simulink model "CustomTelemPX4"  (R2021a)
settings: Solver=FixedStepAuto  StartTime=0.0  StopTime=inf  RelTol=1e-3  EnableMultiTasking=on
InitFcn:
  | Ts = 0.01
libraries: px4uORBlib x4, etargetslib x3, px4lib x1
settings Model: ExtModeTrigDuration=10  Creator=Alireza  LastModifiedBy=Alireza
settings SolverCC: PositivePriorityOrder=on
settings OptimizationCC: EnhancedBackFolding=on  PassReuseOutputArgsAs=Individual arguments  ZeroExternalMemoryAtStartup=off  ZeroInternalMemoryAtStartup=off  MaxStackSize=64  OptimizeBlockOrder=speed  DifferentSizesBufferReuse=on  OptimizationCustomize=off  EfficientTunableParamExpr=on
settings DebuggingCC: ParameterTunabilityLossMsg=error
settings HardwareCC: ProdBitPerPointer=32  ProdBitPerSizeT=32  ProdBitPerPtrDiffT=32  ProdLargestAtomicInteger=Long  ProdLargestAtomicFloat=Double  ProdWordSize=32  ProdLongLongMode=on  ProdHWDeviceType=ARM Compatible->ARM Cortex
settings SFSimCC: MATLABDynamicMemAlloc=off  SimTargetLang=C++
settings RTWCC: SystemTargetFile=ert.tlc  HardwareBoard=PX4 Pixhawk 1  TLCOptions="-aInlineSetEventsForThisBaseRateFcn=TLC_FALSE -aSuppressMultiTaskScheduler=TLC_FALSE  -aRateBasedStepFcn=0"  TemplateMakefile=ert_default_tmf  Toolchain=GNU Tools for PX4 Autopilots  TargetLang=C++
settings CodeAppCC: ForceParamTrailComments=on  IgnoreCustomStorageClasses=off  OperatorAnnotations=on  SimulinkDataObjDesc=on  SFDataObjDesc=on  InsertBlockDesc=on
settings ERTTargetCC: ExtModeTransport=3  ExtModeStaticAlloc=on  ExtModeStaticAllocSize=1024  ExtModeMexFile=ext_xcp  ExtModeIntrfLevel=Level2 - Open

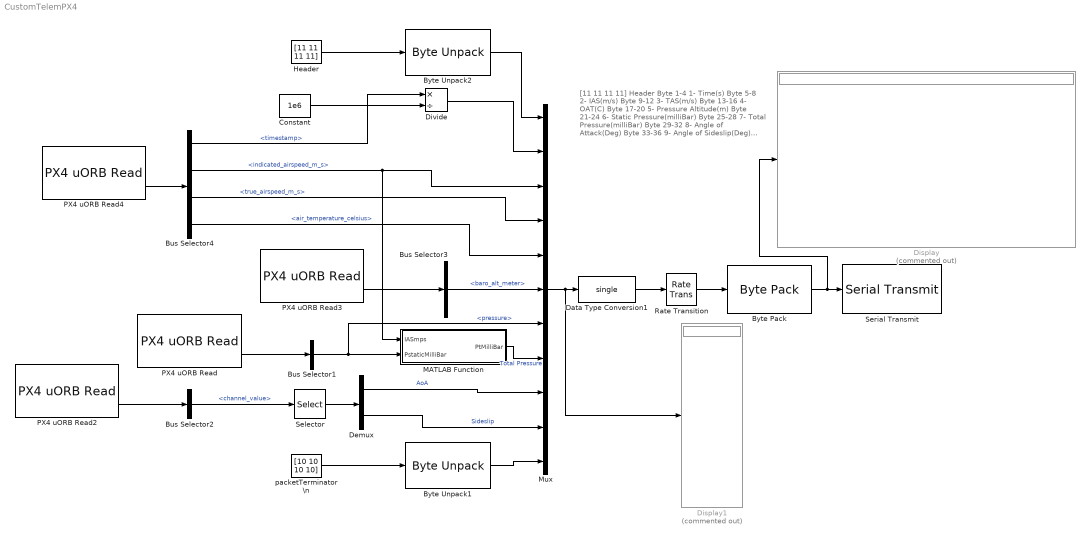
== system CustomTelemPX4 ==
  note: [11 11 11 11] Header Byte 1-4
      | 1- Time(s) Byte 5-8
      | 2- IAS(m/s) Byte 9-12
      | 3- TAS(m/s) Byte 13-16
      | 4- OAT(C) Byte 17-20
      | 5- Pressure Altitude(m) Byte 21-24
      | 6- Static Pressure(milliBar) Byte 25-28
      | 7- Total Pressure(milliBar) Byte 29-32
      | 8- Angle of Attack(Deg) Byte 33-36
      | 9- Angle of Sideslip(Deg) Byte 37-40
      | [10 10 10 10] Terminator Byte 41-44
  Bus Selector1 : BusSelector  OutputSignals=pressure
  Bus Selector2 : BusSelector  OutputSignals=channel_value
  Bus Selector3 : BusSelector  OutputSignals=baro_alt_meter
  Bus Selector4 : BusSelector  OutputSignals=timestamp,indicated_airspeed_m_s,true_airspeed_m_s,air_temperature_celsius
  Byte Pack : etargetslib/Byte Pack  datatypes={'single'}  byteAlign=1
  Byte Unpack1 : etargetslib/Byte Unpack  dimensions={[1]}  datatypes={'single'}  byteAlign=1
  Byte Unpack2 : etargetslib/Byte Unpack  dimensions={[1]}  datatypes={'single'}  byteAlign=1
  Constant : Constant  Value=1e6
  Data Type Conversion1 : DataTypeConversion  OutDataTypeStr=single
  Demux : Demux  Outputs=2
  Display : Display  Commented=on
  Display1 : Display  Commented=on
  Divide : Product  Inputs=*/  OutDataTypeStr=single
  Header : Constant  Value=[11 11 11 11]  OutDataTypeStr=uint8  SampleTime=-1
  MATLAB Function : MATLAB Function  TreatAsAtomicUnit=on
  Mux : Mux  Inputs=11
  PX4 uORB Read : px4uORBlib/PX4 uORB Read  uORBTopic=sensor_baro  selectInstance=sensor_baro  SampleTime=Ts  BlockingMode=off  BlockTimeout=1e-3
      settings: SourceProductBaseCode=PX4AUTOPILOTS
  PX4 uORB Read2 : px4uORBlib/PX4 uORB Read  uORBTopic=adc_report  selectInstance=adc_report  SampleTime=Ts  BlockingMode=off  BlockTimeout=1e-3
      settings: SourceProductBaseCode=PX4AUTOPILOTS
  PX4 uORB Read3 : px4uORBlib/PX4 uORB Read  uORBTopic=vehicle_air_data  selectInstance=vehicle_air_data  SampleTime=Ts  BlockingMode=off  BlockTimeout=1e-3
      settings: SourceProductBaseCode=PX4AUTOPILOTS
  PX4 uORB Read4 : px4uORBlib/PX4 uORB Read  uORBTopic=airspeed  selectInstance=airspeed  SampleTime=Ts  BlockingMode=off  BlockTimeout=1
      settings: SourceProductBaseCode=PX4AUTOPILOTS
  Rate Transition : RateTransition  OutPortSampleTime=0.02
  Selector : Selector  InputPortWidth=12  IndexOptions=Index vector (dialog)  Indices=[7 8]  OutputSizes=1
  Serial Transmit : px4lib/Serial Transmit  SCIModule=/dev/ttyS1
      settings: SourceProductBaseCode=PX4AUTOPILOTS
  packetTerminator \n : Constant  Value=[10 10 10 10]  OutDataTypeStr=uint8  SampleTime=-1
  wires:
  Byte Pack/1 -> Serial Transmit/1, Display/1
  Bus Selector3/1 -> Mux/6  "<baro_alt_meter>"
  Byte Unpack2/1 -> Mux/1
  Demux/1 -> Mux/9  "AoA"
  Bus Selector4/4 -> Mux/5  "<air_temperature_celsius>"
  MATLAB Function/1(PtMilliBar) -> Mux/8  "Total Pressure"
  Byte Unpack1/1 -> Mux/11
  PX4 uORB Read2/2 -> Bus Selector2/1
  PX4 uORB Read3/2 -> Bus Selector3/1
  packetTerminator \n/1 -> Byte Unpack1/1
  Header/1 -> Byte Unpack2/1
  Rate Transition/1 -> Byte Pack/1
  Demux/2 -> Mux/10  "Sideslip"
  PX4 uORB Read4/2 -> Bus Selector4/1
  Bus Selector2/1 -> Selector/1  "<channel_value>"
  Bus Selector4/1 -> Divide/1  "<timestamp>"
  PX4 uORB Read/2 -> Bus Selector1/1
  Bus Selector4/3 -> Mux/4  "<true_airspeed_m_s>"
  Data Type Conversion1/1 -> Rate Transition/1
  Selector/1 -> Demux/1
  Mux/1 -> Display1/1, Data Type Conversion1/1
  Divide/1 -> Mux/2
  Constant/1 -> Divide/2
  Bus Selector4/2 -> MATLAB Function/1(IASmps), Mux/3  "<indicated_airspeed_m_s>"
  Bus Selector1/1 -> Mux/7, MATLAB Function/2(PstaticMilliBar)  "<pressure>"

== matlab function CustomTelemPX4/MATLAB Function ==
  data: IASmps input; PtMilliBar output; PstaticMilliBar input
function PtMilliBar = Ptotal(IASmps,PstaticMilliBar)
ro0 = 1.225;
PtMilliBar = 0.5*ro0*IASmps^2/100 + PstaticMilliBar;
end
